simulink model "TFM_SIMULACI_N1"  (R2023b)
settings: Solver=VariableStepAuto  StartTime=0.0  StopTime=20  RelTol=1e-3
model mask{Gain=0.05, Gain2=0.0223}
  mask prompts: Gain "Vel_Ini"; Gain2 "Coef_Viscoso"
model workspace (MAT data in the model file):
  Gain = 0.05
  Gain2 = 0.0223
values from neighbouring files (symbols this model uses):
  Ts = 0.005    [simulacion_monza_tfm.m]
undefined symbols (not defined in the file or in its folder): DiscIntNeverNeededParam
settings Model: ParameterArgumentNames=Gain,Gain2  Creator=christian  LastModifiedBy=Usuario
settings SolverCC: AlgebraicLoopSolver=TrustRegion
settings DataIOCC: SaveOutput=off  SaveTime=off  ReturnWorkspaceOutputs=off
settings DebuggingCC: UnconnectedInputMsg=warning  UnconnectedOutputMsg=warning  UnconnectedLineMsg=warning  ArithmeticOperatorsInVariantConditions=warning
settings ModelReferenceCC: EnableRefExpFcnMdlSchedulingChecks=on  ModelReferenceNumInstancesAllowed=Single  ModelReferenceMinAlgLoopOccurrences=on
settings SFSimCC: SimUseLocalCustomCode=off  CustomCodeUndefinedFunction=UseInterfaceOnly
settings RTWCC: RTWUseLocalCustomCode=off
settings GRTTargetCC: CombineOutputUpdateFcns=off

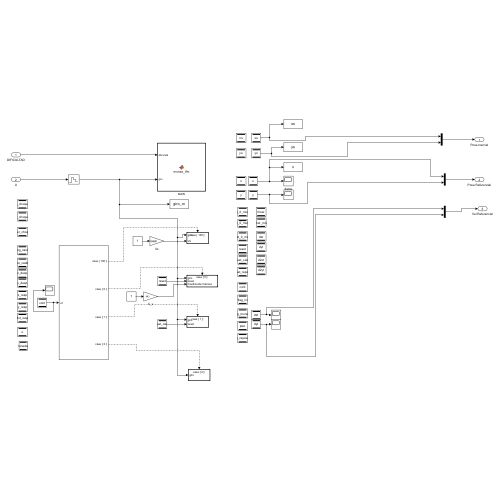
[thumbnail: Simulink's stored preview of the top-level diagram]
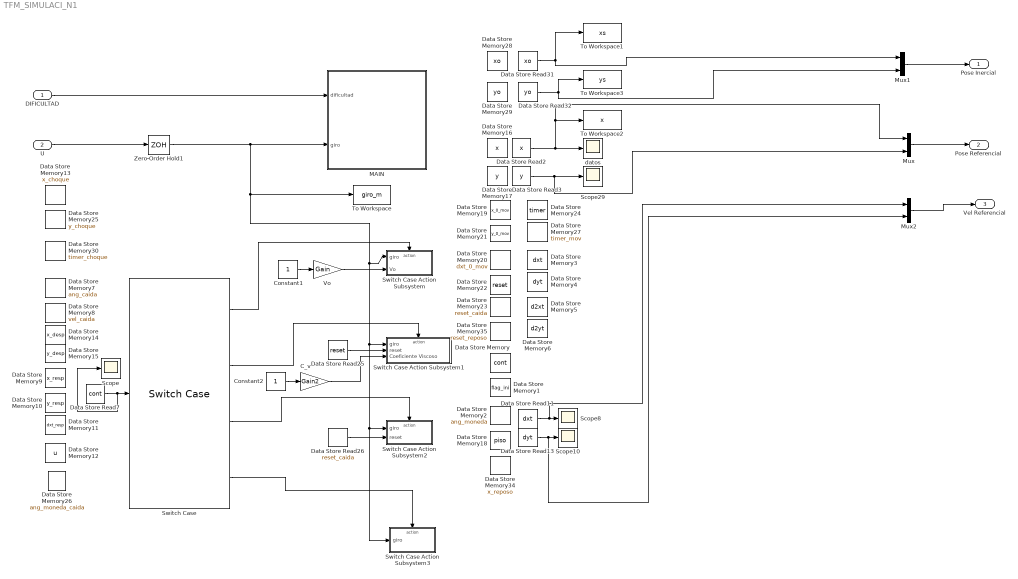
== system TFM_SIMULACI_N1 ==
  DIFICULTAD : Inport  OutDataTypeStr=double  PortDimensions=1
  U : Inport  Port=2  OutDataTypeStr=double  PortDimensions=1  SampleTime=Ts
  C_v : Gain  Gain=Gain2
  Constant1 : Constant
  Constant2 : Constant
  Data Store Memory : DataStoreMemory  DataStoreName=cont  ReadBeforeWriteMsg=warning  WriteAfterWriteMsg=warning  WriteAfterReadMsg=warning  InitialValue=100  ShowAdditionalParam=off  OutDataTypeStr=double
  Data Store Memory1 : DataStoreMemory  DataStoreName=flag_ini  ReadBeforeWriteMsg=warning  WriteAfterWriteMsg=warning  WriteAfterReadMsg=warning  InitialValue=1  ShowAdditionalParam=off  OutDataTypeStr=double
  Data Store Memory10 : DataStoreMemory  DataStoreName=y_resp  ReadBeforeWriteMsg=warning  WriteAfterWriteMsg=warning  WriteAfterReadMsg=warning  ShowAdditionalParam=off  OutDataTypeStr=double
  Data Store Memory11 : DataStoreMemory  DataStoreName=dxt_resp  ReadBeforeWriteMsg=warning  WriteAfterWriteMsg=warning  WriteAfterReadMsg=warning  ShowAdditionalParam=off  OutDataTypeStr=double
  Data Store Memory12 : DataStoreMemory  DataStoreName=u  ReadBeforeWriteMsg=warning  WriteAfterWriteMsg=warning  WriteAfterReadMsg=warning  ShowAdditionalParam=off  OutDataTypeStr=double
  Data Store Memory13 : DataStoreMemory  DataStoreName=x_choque  ReadBeforeWriteMsg=warning  WriteAfterWriteMsg=warning  WriteAfterReadMsg=warning  InitialValue=1  ShowAdditionalParam=off  OutDataTypeStr=double  Dimensions=1
  Data Store Memory14 : DataStoreMemory  DataStoreName=x_desp  ReadBeforeWriteMsg=warning  WriteAfterWriteMsg=warning  WriteAfterReadMsg=warning  ShowAdditionalParam=off  OutDataTypeStr=double
  Data Store Memory15 : DataStoreMemory  DataStoreName=y_desp  ReadBeforeWriteMsg=warning  WriteAfterWriteMsg=warning  WriteAfterReadMsg=warning  ShowAdditionalParam=off  OutDataTypeStr=double
  Data Store Memory16 : DataStoreMemory  DataStoreName=x  ReadBeforeWriteMsg=warning  WriteAfterWriteMsg=warning  WriteAfterReadMsg=warning  InitialValue=-0.11  ShowAdditionalParam=off  OutDataTypeStr=double
  Data Store Memory17 : DataStoreMemory  DataStoreName=y  ReadBeforeWriteMsg=warning  WriteAfterWriteMsg=warning  WriteAfterReadMsg=warning  InitialValue=0.106  ShowAdditionalParam=off  OutDataTypeStr=double
  Data Store Memory18 : DataStoreMemory  DataStoreName=piso  ReadBeforeWriteMsg=warning  WriteAfterWriteMsg=warning  WriteAfterReadMsg=warning  InitialValue=1  ShowAdditionalParam=off  OutDataTypeStr=double
  Data Store Memory19 : DataStoreMemory  DataStoreName=x_0_mov  ReadBeforeWriteMsg=warning  WriteAfterWriteMsg=warning  WriteAfterReadMsg=warning  InitialValue=-0.1206  ShowAdditionalParam=off  OutDataTypeStr=double
  Data Store Memory2 : DataStoreMemory  DataStoreName=ang_moneda  ReadBeforeWriteMsg=warning  WriteAfterWriteMsg=warning  WriteAfterReadMsg=warning  ShowAdditionalParam=off  OutDataTypeStr=double
  Data Store Memory20 : DataStoreMemory  DataStoreName=dxt_0_mov  ReadBeforeWriteMsg=warning  WriteAfterWriteMsg=warning  WriteAfterReadMsg=warning  ShowAdditionalParam=off  OutDataTypeStr=double
  Data Store Memory21 : DataStoreMemory  DataStoreName=y_0_mov  ReadBeforeWriteMsg=warning  WriteAfterWriteMsg=warning  WriteAfterReadMsg=warning  InitialValue=0.106  ShowAdditionalParam=off  OutDataTypeStr=double
  Data Store Memory22 : DataStoreMemory  DataStoreName=reset  ReadBeforeWriteMsg=warning  WriteAfterWriteMsg=warning  WriteAfterReadMsg=warning  ShowAdditionalParam=off  OutDataTypeStr=double
  Data Store Memory23 : DataStoreMemory  DataStoreName=reset_caida  ReadBeforeWriteMsg=warning  WriteAfterWriteMsg=warning  WriteAfterReadMsg=warning  ShowAdditionalParam=off  OutDataTypeStr=double
  Data Store Memory24 : DataStoreMemory  DataStoreName=timer  ReadBeforeWriteMsg=warning  WriteAfterWriteMsg=warning  WriteAfterReadMsg=warning  ShowAdditionalParam=off  OutDataTypeStr=double
  Data Store Memory25 : DataStoreMemory  DataStoreName=y_choque  ReadBeforeWriteMsg=warning  WriteAfterWriteMsg=warning  WriteAfterReadMsg=warning  ShowAdditionalParam=off  OutDataTypeStr=double  Dimensions=1
  Data Store Memory26 : DataStoreMemory  DataStoreName=ang_moneda_caida  ReadBeforeWriteMsg=warning  WriteAfterWriteMsg=warning  WriteAfterReadMsg=warning  ShowAdditionalParam=off  OutDataTypeStr=double
  Data Store Memory27 : DataStoreMemory  DataStoreName=timer_mov  ReadBeforeWriteMsg=warning  WriteAfterWriteMsg=warning  WriteAfterReadMsg=warning  ShowAdditionalParam=off  OutDataTypeStr=double
  Data Store Memory28 : DataStoreMemory  DataStoreName=xo  ReadBeforeWriteMsg=warning  WriteAfterWriteMsg=warning  WriteAfterReadMsg=warning  InitialValue=-0.1  ShowAdditionalParam=off  OutDataTypeStr=double
  Data Store Memory29 : DataStoreMemory  DataStoreName=yo  ReadBeforeWriteMsg=warning  WriteAfterWriteMsg=warning  WriteAfterReadMsg=warning  InitialValue=0.1092  ShowAdditionalParam=off  OutDataTypeStr=double
  Data Store Memory3 : DataStoreMemory  DataStoreName=dxt  ReadBeforeWriteMsg=warning  WriteAfterWriteMsg=warning  WriteAfterReadMsg=warning  ShowAdditionalParam=off  OutDataTypeStr=double
  Data Store Memory30 : DataStoreMemory  DataStoreName=timer_choque  ReadBeforeWriteMsg=warning  WriteAfterWriteMsg=warning  WriteAfterReadMsg=warning  ShowAdditionalParam=off  OutDataTypeStr=double  Dimensions=1
  Data Store Memory34 : DataStoreMemory  DataStoreName=x_reposo  ReadBeforeWriteMsg=warning  WriteAfterWriteMsg=warning  WriteAfterReadMsg=warning  InitialValue=-0.11  ShowAdditionalParam=off  OutDataTypeStr=double
  Data Store Memory35 : DataStoreMemory  DataStoreName=reset_reposo  ReadBeforeWriteMsg=warning  WriteAfterWriteMsg=warning  WriteAfterReadMsg=warning  ShowAdditionalParam=off  OutDataTypeStr=double
  Data Store Memory4 : DataStoreMemory  DataStoreName=dyt  ReadBeforeWriteMsg=warning  WriteAfterWriteMsg=warning  WriteAfterReadMsg=warning  ShowAdditionalParam=off  OutDataTypeStr=double
  Data Store Memory5 : DataStoreMemory  DataStoreName=d2xt  ReadBeforeWriteMsg=warning  WriteAfterWriteMsg=warning  WriteAfterReadMsg=warning  ShowAdditionalParam=off  OutDataTypeStr=double
  Data Store Memory6 : DataStoreMemory  DataStoreName=d2yt  ReadBeforeWriteMsg=warning  WriteAfterWriteMsg=warning  WriteAfterReadMsg=warning  ShowAdditionalParam=off  OutDataTypeStr=double
  Data Store Memory7 : DataStoreMemory  DataStoreName=ang_caida  ReadBeforeWriteMsg=warning  WriteAfterWriteMsg=warning  WriteAfterReadMsg=warning  ShowAdditionalParam=off  OutDataTypeStr=double
  Data Store Memory8 : DataStoreMemory  DataStoreName=vel_caida  ReadBeforeWriteMsg=warning  WriteAfterWriteMsg=warning  WriteAfterReadMsg=warning  ShowAdditionalParam=off  OutDataTypeStr=double
  Data Store Memory9 : DataStoreMemory  DataStoreName=x_resp  ReadBeforeWriteMsg=warning  WriteAfterWriteMsg=warning  WriteAfterReadMsg=warning  ShowAdditionalParam=off  OutDataTypeStr=double
  Data Store Read11 : DataStoreRead  DataStoreName=dxt  IndexOptions=Index vector (dialog)  Indices=1  OutputSizes=1
  Data Store Read13 : DataStoreRead  DataStoreName=dyt  IndexOptions=Index vector (dialog)  Indices=1  OutputSizes=1
  Data Store Read2 : DataStoreRead  DataStoreName=x  IndexOptions=Index vector (dialog)  Indices=1  OutputSizes=1
  Data Store Read25 : DataStoreRead  DataStoreName=reset  IndexOptions=Index vector (dialog)  Indices=1  OutputSizes=1
  Data Store Read26 : DataStoreRead  DataStoreName=reset_caida  IndexOptions=Index vector (dialog)  Indices=1  OutputSizes=1
  Data Store Read3 : DataStoreRead  DataStoreName=y  IndexOptions=Index vector (dialog)  Indices=1  OutputSizes=1
  Data Store Read31 : DataStoreRead  DataStoreName=xo  IndexOptions=Index vector (dialog)  Indices=1  OutputSizes=1
  Data Store Read32 : DataStoreRead  DataStoreName=yo  IndexOptions=Index vector (dialog)  Indices=1  OutputSizes=1
  Data Store Read7 : DataStoreRead  DataStoreName=cont  SampleTime=Ts  IndexOptions=Index vector (dialog)  Indices=1  OutputSizes=1
  MAIN : MATLAB Function  TreatAsAtomicUnit=on  SystemSampleTime=Ts
      settings: MinAlgLoopOccurrences=on
  Mux : Mux  Inputs=2
  Mux1 : Mux  Inputs=2
  Mux2 : Mux  Inputs=2
  Scope{,8,10,29} (4 alike) : Scope
  Switch Case : SwitchCase  CaseConditions={100,0,1,2}  ShowDefaultCase=off
  Switch Case Action Subsystem : Subsystem  TreatAsAtomicUnit=on
  Switch Case Action Subsystem1 : Subsystem  TreatAsAtomicUnit=on
  Switch Case Action Subsystem2 : Subsystem  TreatAsAtomicUnit=on
  Switch Case Action Subsystem3 : Subsystem  TreatAsAtomicUnit=on
  To Workspace : ToWorkspace  VariableName=giro_m  SampleTime=Ts*5
  To Workspace1 : ToWorkspace  VariableName=xs  SampleTime=Ts*5
  To Workspace2 : ToWorkspace  VariableName=x  SampleTime=Ts
  To Workspace3 : ToWorkspace  VariableName=ys  SampleTime=Ts*5
  Vo : Gain  Gain=Gain
  Zero-Order Hold1 : ZeroOrderHold  SampleTime=Ts*10
  datos : Scope
  Pose Inercial : Outport  OutDataTypeStr=double  PortDimensions=2  SampleTime=Ts  VectorParamsAs1DForOutWhenUnconnected=off
  Pose Referencial : Outport  Port=2  OutDataTypeStr=double  PortDimensions=2  SampleTime=Ts  VectorParamsAs1DForOutWhenUnconnected=off
  Vel Referencial : Outport  Port=3  OutDataTypeStr=double  PortDimensions=2  SampleTime=Ts  VectorParamsAs1DForOutWhenUnconnected=off
  wires:
  Vo/1 -> Switch Case Action Subsystem/2(Vo)
  Constant1/1 -> Vo/1
  Data Store Read7/1 -> Scope/1, Switch Case/1
  Data Store Read32/1 -> Mux1/2, To Workspace3/1
  DIFICULTAD/1 -> MAIN/1(dificultad)
  Switch Case/4 -> Switch Case Action Subsystem3/Action
  Data Store Read31/1 -> To Workspace1/1, Mux1/1
  Switch Case/2 -> Switch Case Action Subsystem1/Action
  Data Store Read26/1 -> Switch Case Action Subsystem2/2(reset)
  Switch Case/3 -> Switch Case Action Subsystem2/Action
  Switch Case/1 -> Switch Case Action Subsystem/Action
  U/1 -> Zero-Order Hold1/1
  Data Store Read2/1 -> To Workspace2/1, Mux/1, datos/1
  Data Store Read11/1 -> Scope8/1, Mux2/1
  Data Store Read3/1 -> Scope29/1, Mux/2
  Data Store Read25/1 -> Switch Case Action Subsystem1/2("reset ")
  Data Store Read13/1 -> Scope10/1, Mux2/2
  Constant2/1 -> C_v/1
  C_v/1 -> Switch Case Action Subsystem1/3(Coeficiente Viscoso)
  Mux/1 -> Pose Referencial/1
  Mux1/1 -> Pose Inercial/1
  Mux2/1 -> Vel Referencial/1
  Zero-Order Hold1/1 -> To Workspace/1, Switch Case Action Subsystem/1(giro), Switch Case Action Subsystem1/1(giro), Switch Case Action Subsystem3/1(giro), Switch Case Action Subsystem2/1(giro), MAIN/2(giro)

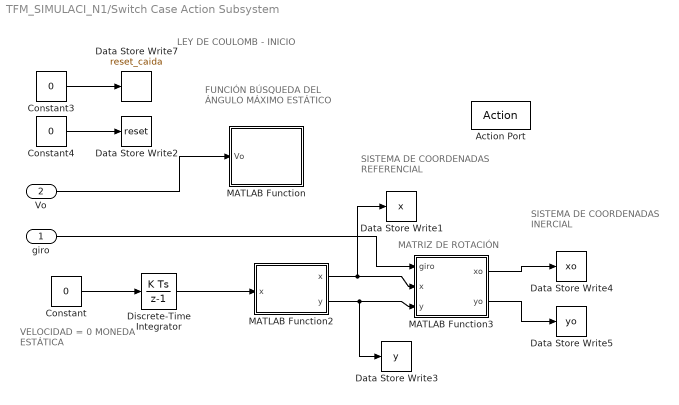
== system TFM_SIMULACI_N1/Switch Case Action Subsystem ==
  note: FUNCIÓN
      | BÚSQUEDA DEL ÁNGULO
      | MÁXIMO ESTÁTICO
  note: LEY DE COULOMB - INICIO
  note: SISTEMA DE
      | COORDENADAS
      | INERCIAL
  note: SISTEMA DE
      | COORDENADAS
      | REFERENCIAL
  note: MATRIZ DE ROTACIÓN
  note: VELOCIDAD = 0
      | MONEDA ESTÁTICA
  giro : Inport  SampleTime=Ts
  Vo : Inport  Port=2
  Action Port : ActionPort  ActionPortLabel=case [ 100 ]:
  Constant : Constant  Value=0
  Constant3 : Constant  Value=0  SampleTime=Ts
  Constant4 : Constant  Value=0  SampleTime=Ts
  Data Store Write1 : DataStoreWrite  DataStoreName=x  SampleTime=Ts  IndexOptions=Index vector (dialog)  Indices=1  OutputSizes=1
  Data Store Write2 : DataStoreWrite  DataStoreName=reset  SampleTime=Ts  IndexOptions=Index vector (dialog)  Indices=1  OutputSizes=1
  Data Store Write3 : DataStoreWrite  DataStoreName=y  SampleTime=Ts  IndexOptions=Index vector (dialog)  Indices=1  OutputSizes=1
  Data Store Write4 : DataStoreWrite  DataStoreName=xo  SampleTime=Ts  IndexOptions=Index vector (dialog)  Indices=1  OutputSizes=1
  Data Store Write5 : DataStoreWrite  DataStoreName=yo  SampleTime=Ts  IndexOptions=Index vector (dialog)  Indices=1  OutputSizes=1
  Data Store Write7 : DataStoreWrite  DataStoreName=reset_caida  SampleTime=Ts  IndexOptions=Index vector (dialog)  Indices=1  OutputSizes=1
  Discrete-Time Integrator : DiscreteIntegrator  InitialCondition=-0.11  SampleTime=Ts  ICPrevOutput=DiscIntNeverNeededParam  ICPrevScaledInput=DiscIntNeverNeededParam
  MATLAB Function : MATLAB Function  TreatAsAtomicUnit=on  SystemSampleTime=Ts
  MATLAB Function2 : MATLAB Function  TreatAsAtomicUnit=on  SystemSampleTime=Ts
  MATLAB Function3 : MATLAB Function  TreatAsAtomicUnit=on  SystemSampleTime=Ts
  wires:
  Constant3/1 -> Data Store Write7/1
  Constant4/1 -> Data Store Write2/1
  MATLAB Function3/2(yo) -> Data Store Write5/1
  MATLAB Function3/1(xo) -> Data Store Write4/1
  MATLAB Function2/2(y) -> Data Store Write3/1, MATLAB Function3/3(y)
  MATLAB Function2/1(x) -> MATLAB Function3/2(x), Data Store Write1/1
  giro/1 -> MATLAB Function3/1(giro)
  Discrete-Time Integrator/1 -> MATLAB Function2/1("x ")
  Constant/1 -> Discrete-Time Integrator/1
  Vo/1 -> MATLAB Function/1(Vo)

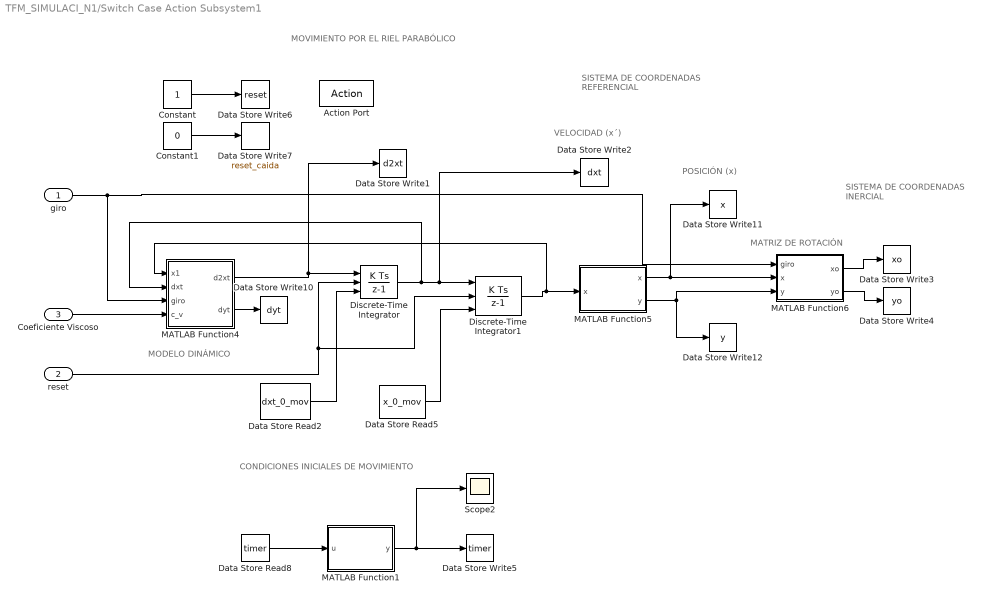
== system TFM_SIMULACI_N1/Switch Case Action Subsystem1 ==
  note: VELOCIDAD (x´)
  note: SISTEMA DE
      | COORDENADAS
      | REFERENCIAL
  note: SISTEMA DE
      | COORDENADAS
      | INERCIAL
  note: MOVIMIENTO POR EL RIEL PARABÓLICO
  note: POSICIÓN (x)
  note: MODELO DINÁMICO
  note: CONDICIONES INICIALES DE MOVIMIENTO
  note: MATRIZ DE ROTACIÓN
  giro : Inport  OutDataTypeStr=double  SampleTime=Ts
  "reset " : Inport  Port=2  OutDataTypeStr=double  SampleTime=Ts
  Coeficiente Viscoso : Inport  Port=3
  Action Port : ActionPort  ActionPortLabel=case [ 0 ]:
  Constant : Constant  SampleTime=Ts
  Constant1 : Constant  Value=0  SampleTime=Ts
  Data Store Read2 : DataStoreRead  DataStoreName=dxt_0_mov  SampleTime=Ts  IndexOptions=Index vector (dialog)  Indices=1  OutputSizes=1
  Data Store Read5 : DataStoreRead  DataStoreName=x_0_mov  SampleTime=Ts  IndexOptions=Index vector (dialog)  Indices=1  OutputSizes=1
  Data Store Read8 : DataStoreRead  DataStoreName=timer  SampleTime=Ts  IndexOptions=Index vector (dialog)  Indices=1  OutputSizes=1
  Data Store Write1 : DataStoreWrite  DataStoreName=d2xt  SampleTime=Ts  IndexOptions=Index vector (dialog)  Indices=1  OutputSizes=1
  Data Store Write10 : DataStoreWrite  DataStoreName=dyt  SampleTime=Ts  IndexOptions=Index vector (dialog)  Indices=1  OutputSizes=1
  Data Store Write11 : DataStoreWrite  DataStoreName=x  SampleTime=Ts  IndexOptions=Index vector (dialog)  Indices=1  OutputSizes=1
  Data Store Write12 : DataStoreWrite  DataStoreName=y  SampleTime=Ts  IndexOptions=Index vector (dialog)  Indices=1  OutputSizes=1
  Data Store Write2 : DataStoreWrite  DataStoreName=dxt  SampleTime=Ts  IndexOptions=Index vector (dialog)  Indices=1  OutputSizes=1
  Data Store Write3 : DataStoreWrite  DataStoreName=xo  SampleTime=Ts  IndexOptions=Index vector (dialog)  Indices=1  OutputSizes=1
  Data Store Write4 : DataStoreWrite  DataStoreName=yo  SampleTime=Ts  IndexOptions=Index vector (dialog)  Indices=1  OutputSizes=1
  Data Store Write5 : DataStoreWrite  DataStoreName=timer  IndexOptions=Index vector (dialog)  Indices=1  OutputSizes=1
  Data Store Write6 : DataStoreWrite  DataStoreName=reset  IndexOptions=Index vector (dialog)  Indices=1  OutputSizes=1
  Data Store Write7 : DataStoreWrite  DataStoreName=reset_caida  SampleTime=Ts  IndexOptions=Index vector (dialog)  Indices=1  OutputSizes=1
  Discrete-Time Integrator : DiscreteIntegrator  ExternalReset=falling  InitialConditionSource=external  InitialCondition=-0.11  SampleTime=Ts  ICPrevOutput=DiscIntNeverNeededParam  ICPrevScaledInput=DiscIntNeverNeededParam
  Discrete-Time Integrator1 : DiscreteIntegrator  ExternalReset=falling  InitialConditionSource=external  InitialCondition=-0.11  SampleTime=Ts  ICPrevOutput=DiscIntNeverNeededParam  ICPrevScaledInput=DiscIntNeverNeededParam
  MATLAB Function1 : MATLAB Function  TreatAsAtomicUnit=on
  MATLAB Function4 : MATLAB Function  TreatAsAtomicUnit=on  SystemSampleTime=Ts
  MATLAB Function5 : MATLAB Function  TreatAsAtomicUnit=on  SystemSampleTime=Ts
  MATLAB Function6 : MATLAB Function  TreatAsAtomicUnit=on  SystemSampleTime=Ts
  Scope2 : Scope
  wires:
  Coeficiente Viscoso/1 -> MATLAB Function4/4(c_v)
  Data Store Read8/1 -> MATLAB Function1/1(u)
  MATLAB Function1/1(y) -> Scope2/1, Data Store Write5/1
  Constant/1 -> Data Store Write6/1
  Constant1/1 -> Data Store Write7/1
  giro/1 -> MATLAB Function6/1(giro), MATLAB Function4/3(giro)
  Discrete-Time Integrator1/1 -> MATLAB Function4/1(x1), MATLAB Function5/1("x ")
  MATLAB Function5/1(x) -> Data Store Write11/1, MATLAB Function6/2(x)
  MATLAB Function5/2(y) -> MATLAB Function6/3(y), Data Store Write12/1
  Discrete-Time Integrator/1 -> Data Store Write2/1, Discrete-Time Integrator1/1, MATLAB Function4/2(dxt)
  MATLAB Function4/1(d2xt) -> Discrete-Time Integrator/1, Data Store Write1/1
  MATLAB Function4/2(dyt) -> Data Store Write10/1
  "reset "/1 -> Discrete-Time Integrator/2, Discrete-Time Integrator1/2
  Data Store Read2/1 -> Discrete-Time Integrator/3
  Data Store Read5/1 -> Discrete-Time Integrator1/3
  MATLAB Function6/1(xo) -> Data Store Write3/1
  MATLAB Function6/2(yo) -> Data Store Write4/1

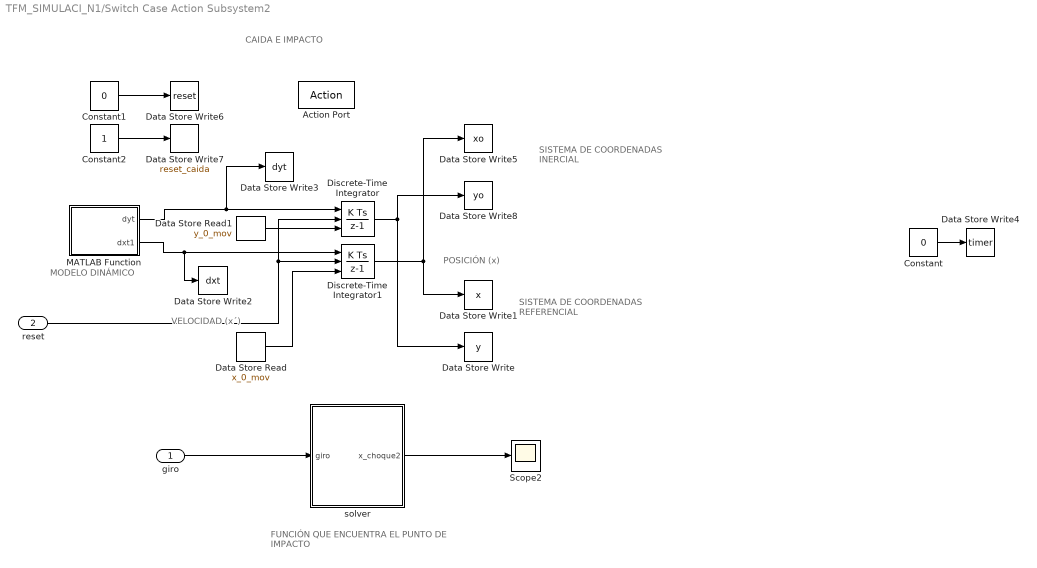
== system TFM_SIMULACI_N1/Switch Case Action Subsystem2 ==
  note: FUNCIÓN QUE
      | ENCUENTRA EL
      | PUNTO DE IMPACTO
  note: CAIDA E IMPACTO
  note: MODELO DINÁMICO
  note: SISTEMA DE
      | COORDENADAS
      | REFERENCIAL
  note: SISTEMA DE
      | COORDENADAS
      | INERCIAL
  note: POSICIÓN (x)
  note: VELOCIDAD (x´)
  giro : Inport  SampleTime=Ts
  reset : Inport  Port=2  SampleTime=Ts
  Action Port : ActionPort  ActionPortLabel=case [ 1 ]:
  Constant : Constant  Value=0  SampleTime=Ts
  Constant1 : Constant  Value=0  SampleTime=Ts
  Constant2 : Constant  SampleTime=Ts
  Data Store Read : DataStoreRead  DataStoreName=x_0_mov  SampleTime=Ts  IndexOptions=Index vector (dialog)  Indices=1  OutputSizes=1
  Data Store Read1 : DataStoreRead  DataStoreName=y_0_mov  SampleTime=Ts  IndexOptions=Index vector (dialog)  Indices=1  OutputSizes=1
  Data Store Write : DataStoreWrite  DataStoreName=y  SampleTime=Ts  IndexOptions=Index vector (dialog)  Indices=1  OutputSizes=1
  Data Store Write1 : DataStoreWrite  DataStoreName=x  SampleTime=Ts  IndexOptions=Index vector (dialog)  Indices=1  OutputSizes=1
  Data Store Write2 : DataStoreWrite  DataStoreName=dxt  SampleTime=Ts  IndexOptions=Index vector (dialog)  Indices=1  OutputSizes=1
  Data Store Write3 : DataStoreWrite  DataStoreName=dyt  SampleTime=Ts  IndexOptions=Index vector (dialog)  Indices=1  OutputSizes=1
  Data Store Write4 : DataStoreWrite  DataStoreName=timer  SampleTime=Ts  IndexOptions=Index vector (dialog)  Indices=1  OutputSizes=1
  Data Store Write5 : DataStoreWrite  DataStoreName=xo  SampleTime=Ts  IndexOptions=Index vector (dialog)  Indices=1  OutputSizes=1
  Data Store Write6 : DataStoreWrite  DataStoreName=reset  SampleTime=Ts  IndexOptions=Index vector (dialog)  Indices=1  OutputSizes=1
  Data Store Write7 : DataStoreWrite  DataStoreName=reset_caida  SampleTime=Ts  IndexOptions=Index vector (dialog)  Indices=1  OutputSizes=1
  Data Store Write8 : DataStoreWrite  DataStoreName=yo  SampleTime=Ts  IndexOptions=Index vector (dialog)  Indices=1  OutputSizes=1
  Discrete-Time Integrator : DiscreteIntegrator  ExternalReset=falling  InitialConditionSource=external  InitialCondition=-0.11  SampleTime=Ts  ICPrevOutput=DiscIntNeverNeededParam  ICPrevScaledInput=DiscIntNeverNeededParam
  Discrete-Time Integrator1 : DiscreteIntegrator  ExternalReset=falling  InitialConditionSource=external  InitialCondition=-0.11  SampleTime=Ts  ICPrevOutput=DiscIntNeverNeededParam  ICPrevScaledInput=DiscIntNeverNeededParam
  MATLAB Function : MATLAB Function  TreatAsAtomicUnit=on  SystemSampleTime=Ts
  Scope2 : Scope
  solver : MATLAB Function  TreatAsAtomicUnit=on  SystemSampleTime=Ts
  wires:
  MATLAB Function/2(dxt1) -> Data Store Write2/1, Discrete-Time Integrator1/1
  MATLAB Function/1(dyt) -> Data Store Write3/1, Discrete-Time Integrator/1
  Data Store Read1/1 -> Discrete-Time Integrator/3
  Discrete-Time Integrator1/1 -> Data Store Write5/1, Data Store Write1/1
  Constant/1 -> Data Store Write4/1
  Data Store Read/1 -> Discrete-Time Integrator1/3
  Constant1/1 -> Data Store Write6/1
  Constant2/1 -> Data Store Write7/1
  Discrete-Time Integrator/1 -> Data Store Write8/1, Data Store Write/1
  giro/1 -> solver/1(giro)
  reset/1 -> Discrete-Time Integrator1/2, Discrete-Time Integrator/2
  solver/1(x_choque2) -> Scope2/1

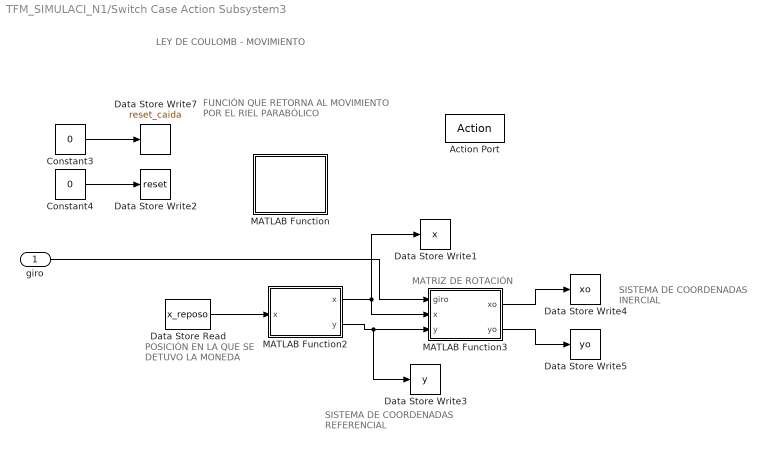
== system TFM_SIMULACI_N1/Switch Case Action Subsystem3 ==
  note: POSICIÓN EN LA
      | QUE SE DETUVO
      | LA MONEDA
  note: MATRIZ DE ROTACIÓN
  note: FUNCIÓN QUE RETORNA
      | AL MOVIMIENTO POR EL
      | RIEL PARABÓLICO
  note: LEY DE COULOMB - MOVIMIENTO
  note: SISTEMA DE
      | COORDENADAS
      | REFERENCIAL
  note: SISTEMA DE
      | COORDENADAS
      | INERCIAL
  giro : Inport  SampleTime=Ts
  Action Port : ActionPort  ActionPortLabel=case [ 2 ]:
  Constant3 : Constant  Value=0  SampleTime=Ts
  Constant4 : Constant  Value=0  SampleTime=Ts
  Data Store Read : DataStoreRead  DataStoreName=x_reposo  SampleTime=Ts  IndexOptions=Index vector (dialog)  Indices=1  OutputSizes=1
  Data Store Write1 : DataStoreWrite  DataStoreName=x  SampleTime=Ts  IndexOptions=Index vector (dialog)  Indices=1  OutputSizes=1
  Data Store Write2 : DataStoreWrite  DataStoreName=reset  SampleTime=Ts  IndexOptions=Index vector (dialog)  Indices=1  OutputSizes=1
  Data Store Write3 : DataStoreWrite  DataStoreName=y  SampleTime=Ts  IndexOptions=Index vector (dialog)  Indices=1  OutputSizes=1
  Data Store Write4 : DataStoreWrite  DataStoreName=xo  SampleTime=Ts  IndexOptions=Index vector (dialog)  Indices=1  OutputSizes=1
  Data Store Write5 : DataStoreWrite  DataStoreName=yo  SampleTime=Ts  IndexOptions=Index vector (dialog)  Indices=1  OutputSizes=1
  Data Store Write7 : DataStoreWrite  DataStoreName=reset_caida  SampleTime=Ts  IndexOptions=Index vector (dialog)  Indices=1  OutputSizes=1
  MATLAB Function : MATLAB Function  TreatAsAtomicUnit=on  SystemSampleTime=Ts
  MATLAB Function2 : MATLAB Function  TreatAsAtomicUnit=on  SystemSampleTime=Ts
  MATLAB Function3 : MATLAB Function  TreatAsAtomicUnit=on  SystemSampleTime=Ts
  wires:
  Data Store Read/1 -> MATLAB Function2/1("x ")
  MATLAB Function2/1(x) -> MATLAB Function3/2(x), Data Store Write1/1
  MATLAB Function3/2(yo) -> Data Store Write5/1
  MATLAB Function3/1(xo) -> Data Store Write4/1
  giro/1 -> MATLAB Function3/1(giro)
  Constant4/1 -> Data Store Write2/1
  MATLAB Function2/2(y) -> Data Store Write3/1, MATLAB Function3/3(y)
  Constant3/1 -> Data Store Write7/1

== matlab function TFM_SIMULACI_N1/Switch Case Action Subsystem/MATLAB Function ==
  settings: updateMethod=DISCRETE
  data: cont data_store_memory; dyt data_store_memory; yo data_store_memory; xo data_store_memory; ang_moneda data_store_memory; flag_ini data_store_memory; dxt data_store_memory; reset data_store_memory; dxt_0_mov data_store_memory; x_0_mov data_store_memory; y_0_mov data_store_memory; d2xt data_store_memory; d2yt data_store_memory; x data_store_memory; reset_reposo data_store_memory; Vo input
function fcn(Vo)
global cont;
global dxt;

global ang_moneda;
global flag_ini;
global reset;
global dxt_0_mov;
global x_0_mov;



if (( flag_ini==1) && (ang_moneda < 0.03)) 
    cont=0;
    x_0_mov=-0.107;
    dxt_0_mov=Vo; %0.05
    reset=0;
else
    cont=100;
    x_0_mov=-0.11;
    dxt=0;
end

== matlab function TFM_SIMULACI_N1/Switch Case Action Subsystem/MATLAB Function2 ==
  settings: updateMethod=DISCRETE
  data: x output; x input; y output
function [x,y] = salida(x)
piso=1;
y=0;
if (piso==1)
    y=-0.54*x^2+0.1143;
else
    if (piso==2)
        y=-0.54*x^2+0.0686;
    else
        if (piso==3)
           y=-0.54*x^2+0.0229; 
        end
    end
end

== matlab function TFM_SIMULACI_N1/Switch Case Action Subsystem/MATLAB Function3 ==
  data: giro input; xo output; x input; y input; yo output
function [xo,yo] = rotacion(giro,x,y)
xo=x*cos(giro)-y*sin(giro);
yo=x*sin(giro)+y*cos(giro);

== matlab function TFM_SIMULACI_N1/Switch Case Action Subsystem1/MATLAB Function1 ==
  data: u input; y output
function y = fcn(u)
y = u+1;

== matlab function TFM_SIMULACI_N1/Switch Case Action Subsystem1/MATLAB Function4 ==
  settings: updateMethod=DISCRETE
  data: x1 input; d2xt output; dxt input; giro input; dyt output; c_v input
function [d2xt,dyt]=fcn(x1,dxt,giro,c_v)
g=9.8;
M=0.007;
c=c_v; %0.01
d2xt=(M*g*-sin(atan(-1.08*x1)+giro)-c*dxt)/(M);
dyt=-1.08*x1*dxt;

== matlab function TFM_SIMULACI_N1/Switch Case Action Subsystem1/MATLAB Function5 ==
  settings: updateMethod=DISCRETE
  data: x output; x input; y output; piso data_store_memory
function [x,y] = salida(x)
global piso;
y=0;
switch piso
    case 1
        y=-0.54*x^2+0.1143;
    case 2
        y=-0.54*x^2+0.0686;
    case 3
        y=-0.54*x^2+0.0229;
    case 4
        y=-0.54*x^2-0.0229;
    case 5
        y=-0.54*x^2-0.0686;
    case 6
        y=-0.54*x^2-0.1143; 
    case 7
        y=-0.54*x^2-0.16;
end

== matlab function TFM_SIMULACI_N1/Switch Case Action Subsystem1/MATLAB Function6 ==
  data: giro input; xo output; x input; y input; yo output
function [xo,yo] = rotacion(giro,x,y)
xo=x*cos(giro)-y*sin(giro);
yo=x*sin(giro)+y*cos(giro);

== matlab function TFM_SIMULACI_N1/Switch Case Action Subsystem2/MATLAB Function ==
  settings: updateMethod=DISCRETE
  data: dyt output; ang_caida data_store_memory; vel_caida data_store_memory; xo data_store_memory; dxt data_store_memory; d2yt data_store_memory; x_resp data_store_memory; dxt1 output; d2xt data_store_memory; x_desp data_store_memory; piso data_store_memory
function [dyt,dxt1]  = caida

global ang_caida;
global vel_caida;
global xo;
global d2yt;
global x_resp;
global d2xt;
global piso;

d2xt=0;
desp=x_resp;
g=9.8;
if (piso ==1 || piso==3 ||piso==5 || piso==7)
    dxt1=vel_caida*(cos(ang_caida));
else
    dxt1=-vel_caida*(cos(ang_caida));
end
dyt=(tan(ang_caida)-((g*(xo))/(vel_caida^2*(cos(ang_caida))^2))+((desp*g)/(vel_caida^2*(cos(ang_caida))^2)))*dxt1; 
d2yt=-g;

== matlab function TFM_SIMULACI_N1/Switch Case Action Subsystem2/solver ==
  settings: updateMethod=DISCRETE
  data: giro input; vel_caida data_store_memory; ang_caida data_store_memory; x_choque data_store_memory; timer_choque data_store_memory; x_desp data_store_memory; y_desp data_store_memory; x_resp data_store_memory; y_resp data_store_memory; piso data_store_memory; y_choque data_store_memory; x_choque2 output
function x_choque2 = fcn(giro)

x_choque2=zeros(4,1);
% y1=0;
coder.extrinsic('solver');
a=cos(giro); b=sin(giro);
global vel_caida;
global ang_caida;
global x_choque;
global y_choque;
global timer_choque;
global x_resp;
global y_resp;
global piso;
timer_choque=timer_choque+1;
[x_choque,y_choque,x_choque2]=solver(a,b,vel_caida,ang_caida,x_resp,y_resp,piso,timer_choque);

== matlab function TFM_SIMULACI_N1/Switch Case Action Subsystem3/MATLAB Function ==
  settings: updateMethod=DISCRETE
  data: ang_moneda data_store_memory; cont data_store_memory; x_0_mov data_store_memory; x data_store_memory; dxt_0_mov data_store_memory; reset data_store_memory; timer_mov data_store_memory
function fcn
global ang_moneda;
global cont;
global x_0_mov;
global x;
global dxt_0_mov;
global reset;
global timer_mov;

if ((ang_moneda < -0.02 || ang_moneda > 0.02))
    cont=0;
    x_0_mov=x;
    dxt_0_mov=0;
    reset=0;
    timer_mov=0;
end

end

== matlab function TFM_SIMULACI_N1/Switch Case Action Subsystem3/MATLAB Function2 ==
  settings: updateMethod=DISCRETE
  data: x output; x input; y output; piso data_store_memory
function [x,y] = salida(x)
global piso;
y=0;
if (piso==1)
    y=-0.54*x^2+0.1143;
else
    if (piso==2)
        y=-0.54*x^2+0.0686;
    else
        if (piso==3)
           y=-0.54*x^2+0.0229; 
        else
           if (piso==4)
                y=-0.54*x^2-0.0229; 
           else
               if (piso==5)
                    y=-0.54*x^2-0.0686;
               else
                   if (piso==6)
                      y=-0.54*x^2-0.1143;
                   else
                       if (piso==7)
                            y=-0.54*x^2-0.16;
                       end
                   end
               end
           end
        end  
    end
end

== matlab function TFM_SIMULACI_N1/Switch Case Action Subsystem3/MATLAB Function3 ==
  data: giro input; xo output; x input; y input; yo output
function [xo,yo] = rotacion(giro,x,y)
xo=x*cos(giro)-y*sin(giro);
yo=x*sin(giro)+y*cos(giro);

== matlab function TFM_SIMULACI_N1/MAIN ==
  settings: updateMethod=DISCRETE
  data: dificultad input; cont data_store_memory; flag_ini data_store_memory; giro input; ang_moneda data_store_memory; vel_caida data_store_memory; ang_caida data_store_memory; x_resp data_store_memory; y_resp data_store_memory; u data_store_memory; x_choque data_store_memory; x_desp data_store_memory; y_desp data_store_memory; piso data_store_memory; x_0_mov data_store_memory; y_0_mov data_store_memory; dxt_0_mov data_store_memory; reset_caida data_store_memory; reset data_store_memory; dyt data_store_memory; ang_moneda_caida data_store_memory; timer_mov data_store_memory; xo data_store_memory; yo data_store_memory; dxt data_store_memory; timer_choque data_store_memory; x_reposo data_store_memory; reset_reposo data_store_memory; x data_store_memory
function monza_tfm(dificultad,giro)
coder.extrinsic('gcs');
coder.extrinsic('set_param');
aux=0;
%*********************VARIABLES GLOBALES**********************************
global cont;
global xo;
global yo;
global ang_moneda;
global flag_ini;
global vel_caida;
global ang_caida;
global ang_moneda_caida;
global x_resp;
global y_resp;
global dyt;
global dxt;
global x_choque;
global x;
global piso;
global x_0_mov;
global y_0_mov;
global dxt_0_mov;
global reset_caida;
global reset;
global reset_reposo;
global timer_mov;
global timer_choque;
global x_reposo;
%*********************ROTACIONES DEL DISCO*********************************
a=cos(giro); 
b=sin(giro);
%*****************INVERSION DEL SENTIDO DE LA u****************************
ang_moneda=atan(-(-b+1.08*a*b*yo+1.08*a^2*xo)/(a+1.08*b^2*yo+1.08*a*b*xo)); 

%***************FINALES DE PISTA**************************************
x1d=0; x2d=0; x3d=0; x4d=0; x5d=0; x6d=0; x7d=0;
x1i=0; x2i=0; x3i=0; x4i=0; x5i=0; x6i=0; x7i=0;

switch dificultad
    case 1
        x1d=0*a-0.11429*b;
        x1i=-0.11*a-0.1092*b;
        
        x2d=0.20646*a-0.04555*b;
        x2i=0*a-0.06857*b;
        
        x3d=0*a-0.02286*b;
        x3i=-0.21142*a+0.00198*b;
        
        x4d=0.20639*a+0.04587*b;
        x4i=0*a+0.02286*b;
        
        x5d=0*a+0.06857*b;
        x5i=-0.19203*a+0.08846*b;
        
        x6d=0.16726*a+0.08757*b;
        x6i=0*a+0.11429*b;
        
        x7d=-0.02554*a+0.16035*b;
        x7i=-0.12744*a+0.16871*b;
        
    case 2
        x1d=0.06211*a-0.11223*b;
        x1i=-0.11*a-0.1092*b;
        
        x2d=0.20646*a-0.04555*b;
        x2i=-0.04758*a-0.06799*b;
        
        x3d=0.04969*a-0.02154*b;
        x3i=-0.21142*a+0.00198*b;
        
        x4d=0.20639*a+0.04587*b;
        x4i=-0.04847*a+0.02411*b;
        
        x5d=0.04406*a+0.06961*b;
        x5i=-0.19203*a+0.08846*b;
        
        x6d=0.16726*a+0.08757*b;
        x6i=-0.05409*a+0.11585*b;
        
        x7d=-0.02554*a+0.16035*b;
        x7i=-0.12744*a+0.16871*b;
    
    case 3
        x1d=0.12394*a-0.10605*b;
        x1i=-0.1*a-0.1092*b;
        
        x2d=0.20646*a-0.04555*b;
        x2i=-0.09503*a-0.06374*b;
        
        x3d=0.09924*a-0.01759*b;
        x3i=-0.21142*a+0.00198*b;
        
        x4d=0.20639*a+0.04587*b;
        x4i=-0.0968*a+0.02787*b;
        
        x5d=0.08803*a+0.07271*b;
        x5i=-0.19203*a+0.08846*b;
        
        x6d=0.16726*a+0.08757*b;
        x6i=-0.108*a+0.12053*b;
        
        x7d=-0.02554*a+0.16035*b;
        x7i=-0.12744*a+0.16871*b;
        
     case 4
        x1d=0.12394*a-0.10605*b;
        x1i=-0.1*a-0.1092*b;
        
        x2d=0.20646*a-0.04555*b;
        x2i=-0.14224*a-0.05771*b;
        
        x3d=0.14851*a-0.01102*b;
        x3i=-0.21142*a+0.00198*b;
        
        x4d=0.20639*a+0.04587*b;
        x4i=-0.14488*a+0.03412*b;
        
        x5d=0.1318*a+0.07789*b;
        x5i=-0.19203*a+0.08846*b;
        
        x6d=0.16726*a+0.08757*b;
        x6i=-0.108*a+0.12053*b;
        
        x7d=-0.02554*a+0.16035*b;
        x7i=-0.12744*a+0.16871*b;
        
        
end


if cont==0
	reset_caida=0;
    reset_reposo=0;
    timer_mov=timer_mov+1;
    switch piso
        case 1
            if xo>=(x1d)
                cont=1;
                aux=1;
                reset_caida=0;
            else
                if ( (xo<=x1i) )
%                 if giro>0
                    if timer_mov>10
                        cont=100;
                        timer_mov=0;
                    end
                    flag_ini=1;
                    reset=0;
                else
                    flag_ini=0;
                end
            end
        case 2
            if xo<=(x2i)
                cont=1;
                aux=1;
                reset_caida=0;                
            else
                if xo>(x2d)
                    set_param(gcs, 'SimulationCommand', 'stop')
                end
            end
        case 3
            if xo>=(x3d)
                cont=1;
                aux=1;
                reset_caida=0;                
            else
                if xo<(x3i)
                    set_param(gcs, 'SimulationCommand', 'stop')
                end
            end
        case 4
            if xo<=(x4i)
                cont=1;
                aux=1;
                reset_caida=0;                
            else
                if xo>(x4d)
                    set_param(gcs, 'SimulationCommand', 'stop')
                end
            end
         case 5
            if xo>=(x5d)
                cont=1;
                aux=1;
                reset_caida=0;                
            else
                if xo<(x5i)
                    set_param(gcs, 'SimulationCommand', 'stop')
                end
            end
         case 6
            if xo<=(x6i)
                cont=1;
                aux=1;
                reset_caida=0;                
            else
                if xo>(x6d)
                    set_param(gcs, 'SimulationCommand', 'stop')
                end
            end
         case 7
            if xo>=(x7i) || xo<(x7d) 
                set_param(gcs, 'SimulationCommand', 'stop')
            end
            
    end
    
    if aux==1
        vel_caida=sqrt(dxt^2+dyt^2);
        ang_caida=ang_moneda;
        x_resp=xo;
        y_resp=yo;
        x_0_mov=xo;
        y_0_mov=yo;
%         reset_caida=1;
    end
    if ((dxt>-0.02) && (dxt<0.02) && (a*xo+b*yo)>(x1i+0.02) && ((ang_moneda<0.01 && ang_moneda>-0.01)))
        cont=2;
        x_reposo=a*xo+b*yo;
    end
else
    if cont==1
        reset_caida=1;
        ang_moneda_caida=atan(tan(ang_caida)-(9.8*(xo-x_resp))/(vel_caida^2*(cos(ang_caida))^2));
        if ((xo>=x_choque) && (piso==1 || piso==3 || piso==5 || piso==7))
            cont=0;
            piso=piso+1;
            x_0_mov=a*xo+b*yo;
            y_0_mov=a*yo-b*xo;
            dxt_0_mov=sqrt(dxt^2+dyt^2)*cos(-ang_moneda_caida+giro);
            timer_choque=0;
            reset=0;
        else
            if ((xo<=x_choque) && (piso==2 || piso==4 || piso==6))
                cont=0;
                piso=piso+1;
                x_0_mov=a*xo+b*yo;
                y_0_mov=a*yo-b*xo;
                dxt_0_mov=-sqrt(dxt^2+dyt^2)*cos(ang_moneda_caida-giro);
                timer_choque=0;
                reset=0;
            end
        end

    end
end
